simulink model "01_ee_a"  (R2023a)
settings: Solver=VariableStepDiscrete  StartTime=0.0  StopTime=6  RelTol=1e-3  EnableMultiTasking=on
PreLoadFcn:
  | %DFIG Data
  | clear;
  | NumberOfDFIG=100;
  | PnomDFIG=2e6*NumberOfDFIG; % Nominal power of DFIG(VA)
  | VnomDFIG=690;       % Line-Line voltage (Vrms)
  | fnom=50;
  | Rs=0.0108;     %pu
  | Lls=0.102;      %pu
  | Rr=0.01021;       %pu
  | Llr=0.11;      %pu
  | Lm=3.362;         %pu
  | Hg=2;         %Inertia constant (s)
  | F=0.01;         %Friction factor (pu)
  | p=2;            %Number of pairs of poles
  | kt=3;     %Rotor/Stator turns rotio
  | slip=-0.1;
  | 
  | %DC link
  | Vdc_nom=1200;       %Volts
  | C_DClink=15000e-6*NumberOfDFIG; %Farads
  | 
  | %Choke data
  | R_RL=0.15/100;  %pu
  | L_RL=0.15;      %pu
InitFcn:
  | Ts_Power = 10e-6;
  | Ts_Control = 100e-6;
  | PWM_freq=50*40;
undefined symbols (not defined in the file): D1, Delta, DiscIntNeverNeededParam
libraries: powerlib_extras x23, spsThreePhaseVIMeasurementLib x4, simulink_extras x4, spsThreePhaseTransformerTwoWindingsLib x2, spsUniversalBridgeLib x2, spsThreePhaseSeriesRLCBranchLib x2, spsParallelRLCBranchLib x1, spsThreePhaseProgrammableVoltageSourceLib x1, spsAsynchronousMachinepuUnitsLib x1, spsThreePhaseSeriesRLCLoadLib x1, spsGroundLib x1, spsMultimeterLib x1
(part 1 of 2)
settings Model: SimulationMode=accelerator  Creator=eagleyi  LastModifiedBy=eagle
settings SolverCC: AlgebraicLoopSolver=TrustRegion
settings DataIOCC: LimitDataPoints=on  SaveFormat=StructureWithTime  SignalLoggingSaveFormat=ModelDataLogs  ReturnWorkspaceOutputs=off
settings OptimizationCC: ExpressionDepthLimit=2147483647  InitFltsAndDblsToZero=on  LifeSpan=inf
settings DebuggingCC: UnderspecifiedInitializationDetection=Classic  MergeDetectMultiDrivingBlocksExec=none  SolverPrmCheckMsg=warning  FcnCallInpInsideContextMsg=warning  UnconnectedInputMsg=warning  UnconnectedOutputMsg=warning  UnconnectedLineMsg=warning  StateNameClashWarn=warning  SFUnexpectedBacktrackingDiag=warning  SFNoUnconditionalDefaultTransitionDiag=warning  SFExecutionAtInitializationDiag=none  ArithmeticOperatorsInVariantConditions=warning
settings HardwareCC: ProdBitPerPointer=32  ProdBitPerSizeT=32  ProdBitPerPtrDiffT=32  ProdLargestAtomicFloat=None  ProdIntDivRoundTo=Undefined  ProdEndianess=Unspecified  ProdWordSize=32  ProdHWDeviceType=32-bit Generic
settings ModelReferenceCC: PropagateSignalLabelsOutOfModel=off
settings SFSimCC: SimUseLocalCustomCode=off  CustomCodeUndefinedFunction=UseInterfaceOnly
settings RTWCC: RTWUseLocalCustomCode=off
settings CodeAppCC: StateflowObjectComments=on
settings GRTTargetCC: TargetLangStandard=C89/C90 (ANSI)  CombineOutputUpdateFcns=off  GRTInterface=on
settings ConfigComp: CovMetricSettings=dw  CovSaveCumulativeToWorkspaceVar=on  CovSaveSingleToWorkspaceVar=on  CovExternalEMLEnable=off  CovSFcnEnable=off
settings SimscapeCC: SimscapeNormalizeSystem=off

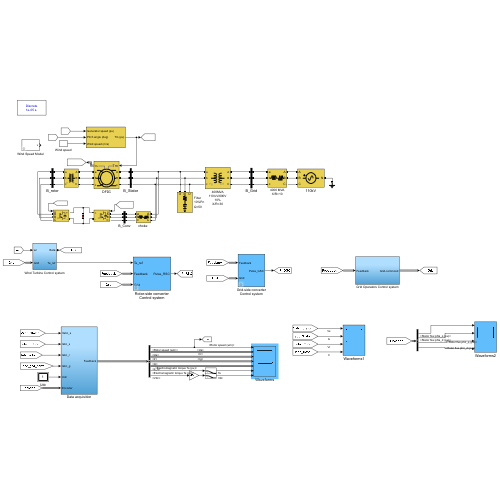
[thumbnail: Simulink's stored preview of the top-level diagram]
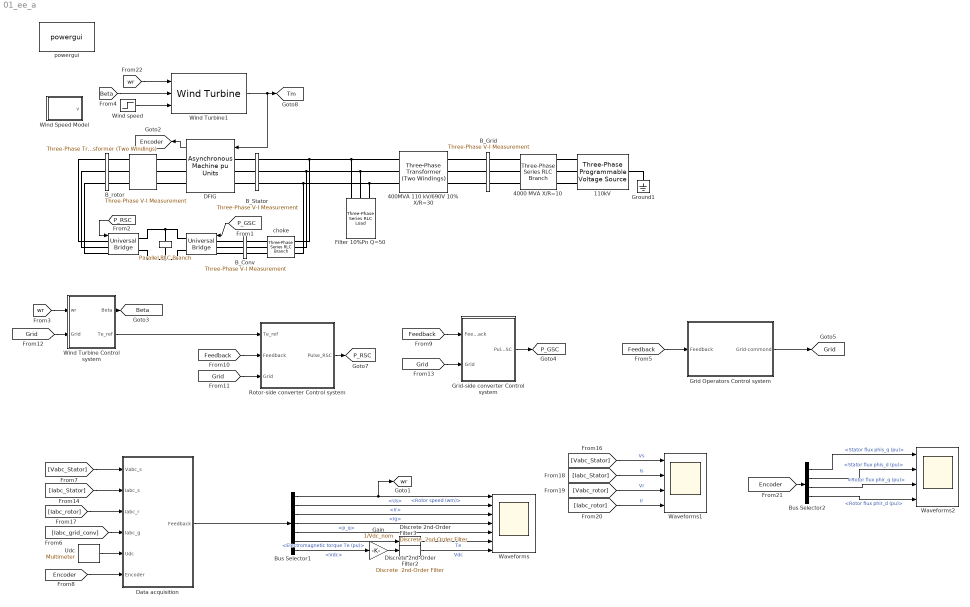
== system 01_ee_a ==
  " " : spsParallelRLCBranchLib/Parallel RLC Branch  LConnTagsString=a  RConnTagsString=__new0  BranchType=C  Resistance=1000  Inductance=1e-3  SetiL0=off  InitialCurrent=0  Capacitance=C_DClink  Setx0=on  InitialVoltage=Vdc_nom  Measurements=Branch voltage
  "  " : spsThreePhaseTransformerTwoWindingsLib/Three-Phase Transformer (Two Windings)  Winding1Connection=Y  Winding2Connection=Y  CoreType=Three single-phase transformers  SetSaturation=off  Hysteresis=off  DataFile='basic_model'  SetInitialFlux=off  Measurements=None  UNITS=pu  NominalPower=[PnomDFIG*0.3 5 ]  Winding1="[ VnomDFIG*0.25  0   0]"  Winding2="[VnomDFIG*0.25*kt  0  0.0001]"  Rm=500  Lm=500  L0=0.5  Saturation="[ 0,0  ;  0.005,1.2  ;  1.0,1.4 ]"  InitialFluxes=[ 0.8 , -0.8 , 0.7 ]  BreakLoop=off  DiscreteSolver=Trapezoidal iterative  DataType=off  TransfoNumber=0
  "   " : spsUniversalBridgeLib/Universal Bridge  Arms=3  SnubberResistance=1e5  SnubberCapacitance=inf  Device=IGBT / Diodes  Ron=1e-5  Lon=0  ForwardVoltages="[  0  0  ]"  ForwardVoltage=0  GTOparameters=[ 10e-6 , 20e-6 ]  IGBTparameters=[ 0 , 0 ]  Measurements=None  Measurements_2=None  converterType=Rectifier
  "          " : spsUniversalBridgeLib/Universal Bridge  Arms=3  SnubberResistance=1e5  SnubberCapacitance=inf  Device=IGBT / Diodes  Ron=1e-5  Lon=0  ForwardVoltages="[  0  0  ]"  ForwardVoltage=0  GTOparameters=[ 10e-6 , 20e-6 ]  IGBTparameters=[ 0 , 0 ]  Measurements=None  Measurements_2=None  converterType=Rectifier
  110kV : spsThreePhaseProgrammableVoltageSourceLib/Three-Phase Programmable Voltage Source  PositiveSequence=[110e3 0 fnom]  VariationEntity=Amplitude  VariationType=Table of time-amplitude pairs  VariationTypeAlt=Step  VariationStep=-0.2  VariationRate=10  VariationMagnitude=0.3  VariationFrequency=2  VariationTiming=[0.05 0.05+5/60]  VariationPhaseA=off  Amplitudes=[1 0.4 1.0]  TimeValues=[0 5 5.625]  HarmonicGeneration=off  HarmonicA=[1 0 0 2]  HarmonicB=[0 0 0 0]  Timing="[1  20]"  BusType=swing  Pref=0  Qref=0  Qmin=-inf  Qmax=inf
  4000 MVA X/R=10 : spsThreePhaseSeriesRLCBranchLib/Three-Phase Series RLC Branch  LConnTagsString=A|B|C  RConnTagsString=A|B|C  BranchType=RL  Resistance=0.1*110^2/4000  Inductance=1/(2*pi*50)*110^2/4000  Capacitance=1.0  Measurements=None
  400MVA 110 kV/690V 10% X/R=30 : spsThreePhaseTransformerTwoWindingsLib/Three-Phase Transformer (Two Windings)  Winding1Connection=Delta (D1)  Winding2Connection=Yg  CoreType=Three single-phase transformers  SetSaturation=off  Hysteresis=off  DataFile='basic_model'  SetInitialFlux=off  Measurements=None  UNITS=pu  NominalPower=[400e6 fnom ]  Winding1="[ 110e3  0.05/30   0.05]"  Winding2="[ 690 0.05/30  0.05]"  Rm=500  Lm=500  L0=0.5  Saturation="[ 0,0  ;  0.005,1.2  ;  1.0,1.4 ]"  InitialFluxes=[ 0.8 , -0.8 , 0.7 ]  BreakLoop=off  DiscreteSolver=Trapezoidal iterative  DataType=off  TransfoNumber=0
  B_Conv : spsThreePhaseVIMeasurementLib/Three-Phase V-I Measurement  VoltageMeasurement=no  SetLabelV=on  LabelV=Vabc_grid_conv  Vpu=off  VpuLL=off  CurrentMeasurement=yes  SetLabelI=on  LabelI=Iabc_grid_conv  Ipu=on  Pbase=PnomDFIG  Vbase=VnomDFIG  OutputType=Complex  PhasorSimulation=off  PSBequivalent=0
  B_Grid : spsThreePhaseVIMeasurementLib/Three-Phase V-I Measurement  VoltageMeasurement=no  SetLabelV=on  LabelV=Vabc_B6  Vpu=on  VpuLL=off  CurrentMeasurement=no  SetLabelI=on  LabelI=Iabc_B4  Ipu=on  Pbase=Pnom  Vbase=115e3  OutputType=Complex  PhasorSimulation=off  PSBequivalent=0
  B_Stator : spsThreePhaseVIMeasurementLib/Three-Phase V-I Measurement  VoltageMeasurement=phase-to-ground  SetLabelV=on  LabelV=Vabc_Stator  Vpu=on  VpuLL=off  CurrentMeasurement=yes  SetLabelI=on  LabelI=Iabc_Stator  Ipu=on  Pbase=PnomDFIG  Vbase=VnomDFIG  OutputType=Complex  PhasorSimulation=off  PSBequivalent=0
  B_rotor : spsThreePhaseVIMeasurementLib/Three-Phase V-I Measurement  VoltageMeasurement=phase-to-phase  SetLabelV=on  LabelV=Vabc_rotor  Vpu=on  VpuLL=off  CurrentMeasurement=yes  SetLabelI=on  LabelI=Iabc_rotor  Ipu=on  Pbase=PnomDFIG  Vbase=VnomDFIG*3  OutputType=Complex  PhasorSimulation=off  PSBequivalent=0
  Bus Selector1 : BusSelector  OutputSignals=Power&Torque&Speed.Rotor speed (wm),Synchronous Frame.Us,Synchronous Frame.Ir,Synchronous Frame.Ig,Power&Torque&Speed.p&q_stator.p_q,Power&Torque&Speed.Electromagnetic torque Te (pu),Stationary Frame.Vdc
  Bus Selector2 : BusSelector  OutputSignals=Stator measurements.Stator flux phis_q (pu),Stator measurements.Stator flux phis_d (pu),Rotor measurements.Rotor flux phir_q (pu),Rotor measurements.Rotor flux phir_d (pu)
  DFIG : spsAsynchronousMachinepuUnitsLib/Asynchronous Machine pu Units  RotorType=Wound  PresetModel=No  MechanicalLoad=Torque Tm  ShowDetailedParameters=on  ReferenceFrame=Synchronous  Units=pu  MeasurementBus=off  NominalParameters=[PnomDFIG VnomDFIG fnom]  VoltageRatio=1  Stator=[Rs Lls]  Rotor=[Rr Llr]  Cage1=[0.01909 0.0397]  Cage2=[0.01909 0.0397]  Lm=Lm  Mechanical=[Hg F p]  PolePairs=2  InitialConditions="[ slip, 0   0,0,0   0,0,0 ]"  SimulateSaturation=off  Saturation="[0.212,0.4201,0.8125,1.0979,1.4799,2.2457,3.2586,4.5763,6.4763 ;   0.5,0.7,0.9,1,1.1,1.2 ,1.3,1.4,1.5]"  LoadFlowParameters=0  TsPowergui=0  TsBlock=-1  IterativeModel=Forward Euler  IterativeDiscreteModel=Trapezoidal non iterative  Pmec=0
      settings: LibrarySourceBlock=|
      | sps_lib/Electrical Machines/Asynchronous Machine
      | pu Units
  Data acquisition : Subsystem
  Discrete 2nd-Order Filter2 : powerlib_extras/Discrete  Control Blocks/Discrete  2nd-Order Filter  FilterType=Lowpass  Fo=1000  Zeta=0.707  Ts=Ts_Power  Initialize=off  Vac_Init=[0.8 -25 60]  Vdc_Init=-0.4  PlotResponse=off  param1=[1 5000 10]
  Discrete 2nd-Order Filter3 : powerlib_extras/Discrete  Control Blocks/Discrete  2nd-Order Filter  FilterType=Lowpass  Fo=1000  Zeta=0.707  Ts=Ts_Power  Initialize=off  Vac_Init=[0.8 -25 60]  Vdc_Init=-0.4  PlotResponse=off  param1=[1 5000 10]
  Filter 10%Pn Q=50 : spsThreePhaseSeriesRLCLoadLib/Three-Phase Series RLC Load  LConnTagsString=A|B|C  Configuration=Y (grounded)  NominalVoltage=VnomDFIG  Vabc=[1e3 1e3 1e3]  Vabcp=[1e3 1e3 1e3]  NominalFrequency=fnom  UnbalancedPower=off  ActivePower=PnomDFIG*0.1/50  InductivePower=0  CapacitivePower=PnomDFIG*0.1  Pabc=[10e3 9e3 11e3]  QLabc=[100 90 110]  QCabc=[100 90 110]  Pabcp=[10e3 9e3 11e3]  QLabcp=[100 90 110]  QCabcp=[100 90 110]  Measurements=None  LoadType=constant Z
  Gain : Gain  Gain=1/Vdc_nom
  Grid Operators Control system : Subsystem
  Grid-side converter Control system : Subsystem  mask{Kpi_grid_side=[0.5 100 1], Kpi_DC_voltage=[2 20 0.5]}
      mask prompts: Kpi_grid_side "PI controller of Grid-side Current"; Kpi_DC_voltage "PI controller of DC Voltage"
      mask init:
      | Kp_grid_side_cur_reg=Kpi_grid_side(1);
      | Ki_grid_side_cur_reg=Kpi_grid_side(2);
      | Limit_U_grid_side=Kpi_grid_side(3);
      | Kp_dc_reg=Kpi_DC_voltage(1);
      | Ki_dc_reg=Kpi_DC_voltage(2);
      | Imax_grid_conv=Kpi_DC_voltage(3);
  Ground1 : spsGroundLib/Ground  LConnTagsString=a
  Rotor-side converter Control system : Subsystem  mask{KQ=[0.5 100 1], K_Irp=[0.5 100 1]}
      mask prompts: KQ "Reactive Power Controller [Kp Ki Limit]"; K_Irp "Rotor Curretnt Controller [Kp Ki Limit]"
      mask init:
      | Kp_Q=KQ(1);
      | Ki_Q=KQ(2);
      | Limit_Q=KQ(3);
      | Kp_rotor_side_cur_reg_P=K_Irp(1);
      | Ki_rotor_side_cur_reg_P=K_Irp(2);
      | Limit_U=K_Irp(3);
  Udc : spsMultimeterLib/Multimeter  L=1  sel=1  yselected={}  Gain=1  OutputType=Complex  PlotAtSimulationStop=off  PhasorSimulation=off
  Waveforms : Scope  NumInputPorts=7
  Waveforms1 : Scope  NumInputPorts=4
  Waveforms2 : Scope  NumInputPorts=4
  Wind Speed Model : Subsystem  mask{Vav=8, Vte=[5 10 3], Vgr=[5 35 2], Vnmax=1}
      mask prompts: Vav "Average wind speed"; Vte "Terbulent wind [tg1  Tg  Vgmax]"; Vgr "Gradual wind [tr1 tr2 Vrmax]"; Vnmax "Random wind Vrmax"
      mask init:
      | tg1=Vte(1);
      | Tg=Vte(2);
      | Vgmax=Vte(3);
      | tr1=Vgr(1);
      | tr2=Vgr(2);
      | Vrmax=Vgr(3);
  Wind Turbine Control system : Subsystem
  Wind Turbine1 : spsWindTurbineLib/Wind Turbine  Pnom=PnomDFIG  Pelec_base=PnomDFIG  wind_base=12  P_wind_base=1  speed_nom=1.1  pitch_angle=0  c1_c6="[0.51763          116          0.4            5           21     0.006795]"  cp_nom=0.48  lambda_nom=8.1
  Wind speed : Step  Time=4  Before=12  After=12  SampleTime=0
  "choke " : spsThreePhaseSeriesRLCBranchLib/Three-Phase Series RLC Branch  LConnTagsString=A|B|C  RConnTagsString=A|B|C  BranchType=RL  Resistance=R_RL*VnomDFIG^2/(0.1*PnomDFIG)  Inductance=L_RL*VnomDFIG^2/(0.1*PnomDFIG)/(2*pi*fnom)  Capacitance=[]  Measurements=None
  powergui : sps_lib/powergui  Priority=2  SimulationMode=Discrete  SampleTime=Ts_Power  frequency=60  Iterations=50  frequencyindice=0  Pbase=100e6  ErrMax=1e-4  UnitsV=kV  UnitsW=MW  buscounter=0  FunctionMessages=off  echomessages=on  EnableUseOfTLC=off  CurrentSourceSwitches=off  DisableSnubberDevices=off  DisableRonSwitches=off  DisableVfSwitches=off  DisplayEquations=off  AutomaticDiscreteSolvers=off  SolverType=Tustin  Interpol=off  ExternalGateDelay=off  methode=off  Ts=0  x0status=blocks  SPID=off  SwTol=0  HookPort=off  NonlinearTolerance=1e-4  nMaxIteration=100  ContinueOnMaxIteration=off  RestoreLinks=warning  ResistiveCurrentMeasurement=off  Frange=[0:2:500]  Ylog=off  Xlog=on  ShowGrid=off  save=off  variable=ZData  structure=ScopeData1  ZoomFFT=off  StartTime=1.4  cycles=1  DisplayStyle=1  fundamental=50  FreqAxis=off  MaxFrequency=500  frequencyindicesteady=1  RmsSteady=1  display=off
  tag scope: Beta=global, Encoder=global, Grid=global, P_GSC=global, P_RSC=global, Tm=global, wr=global
  wires:
  DFIG/1 -> [Encoder]
  [P_GSC] -> "          "/1
  [P_RSC] -> "   "/1
  Bus Selector1/4 -> Waveforms/4  "<Ig>"
  Bus Selector1/1 -> [wr], Waveforms/1  "<Rotor speed (wm)>"
  Bus Selector1/2 -> Waveforms/2  "<Us>"
  Bus Selector1/3 -> Waveforms/3  "<Ir>"
  Bus Selector1/5 -> Waveforms/5  "<p_q>"
  Bus Selector1/6 -> Discrete 2nd-Order Filter2/1  "<Electromagnetic torque Te (pu)>"
  Bus Selector1/7 -> Gain/1  "<Vdc>"
  Gain/1 -> Discrete 2nd-Order Filter3/1
  Discrete 2nd-Order Filter2/1 -> Waveforms/6  "Te"
  Discrete 2nd-Order Filter3/1 -> Waveforms/7  "Vdc"
  Wind Turbine Control system/1(Beta) -> [Beta]
  Grid-side converter Control system/1(Pulse_GSC) -> [P_GSC]
  [Vabc_Stator] -> Data acquisition/1(Vabc_s)
  [Iabc_Stator] -> Data acquisition/2(Iabc_s)
  [Iabc_rotor] -> Data acquisition/3(Iabc_r)
  Udc/1 -> Data acquisition/5(Udc)
  [Iabc_grid_conv] -> Data acquisition/4(Iabc_g)
  [Encoder] -> Data acquisition/6(Encoder)
  Data acquisition/1(Feedback) -> Bus Selector1/1
  Rotor-side converter Control system/1(Pulse_RSC) -> [P_RSC]
  Wind Turbine Control system/2(Te_ref) -> Rotor-side converter Control system/1(Te_ref)
  [Feedback] -> Grid-side converter Control system/1(Feedback)
  [Feedback] -> Rotor-side converter Control system/2(Feedback)
  [wr] -> Wind Turbine Control system/1(wr)
  [Grid] -> Rotor-side converter Control system/3(Grid)
  Grid Operators Control system/1(Grid-commond) -> [Grid]
  [Grid] -> Wind Turbine Control system/2(Grid)
  [Grid] -> Grid-side converter Control system/2(Grid)
  Wind Turbine1/1 -> DFIG/1, [Tm]
  [Feedback] -> Grid Operators Control system/1(Feedback)
  Wind speed/1 -> Wind Turbine1/3
  [Vabc_Stator] -> Waveforms1/1  "Vs"
  [Iabc_Stator] -> Waveforms1/2  "Is"
  [Vabc_rotor] -> Waveforms1/3  "Vr"
  [Iabc_rotor] -> Waveforms1/4  "Ir"
  [Encoder] -> Bus Selector2/1
  Bus Selector2/4 -> Waveforms2/4  "<Rotor flux phir_d (pu)>"
  Bus Selector2/1 -> Waveforms2/1  "<Stator flux phis_q (pu)>"
  Bus Selector2/2 -> Waveforms2/2  "<Stator flux phis_d (pu)>"
  Bus Selector2/3 -> Waveforms2/3  "<Rotor flux phir_q (pu)>"
  [wr] -> Wind Turbine1/1
  [Beta] -> Wind Turbine1/2
  connections:
  "   "/RConn1 -- " "/LConn1 -- "          "/RConn1
  "          "/RConn2 -- " "/RConn1 -- "   "/RConn2
  B_Stator/LConn1 -- Filter 10%Pn Q=50/LConn1 -- 400MVA 110 kV/690V 10% X/R=30/RConn1 -- "choke "/LConn1
  B_Stator/LConn2 -- Filter 10%Pn Q=50/LConn2 -- 400MVA 110 kV/690V 10% X/R=30/RConn2 -- "choke "/LConn2
  B_Stator/LConn3 -- Filter 10%Pn Q=50/LConn3 -- 400MVA 110 kV/690V 10% X/R=30/RConn3 -- "choke "/LConn3
  DFIG/LConn2 -- B_Stator/RConn2
  B_Conv/LConn2 -- "choke "/RConn2
  DFIG/LConn3 -- B_Stator/RConn3
  DFIG/LConn1 -- B_Stator/RConn1
  "          "/LConn3 -- B_Conv/RConn3
  B_Conv/LConn3 -- "choke "/RConn3
  "          "/LConn2 -- B_Conv/RConn2
  B_rotor/LConn2 -- "   "/LConn2
  B_rotor/LConn3 -- "   "/LConn3
  B_rotor/LConn1 -- "   "/LConn1
  "          "/LConn1 -- B_Conv/RConn1
  B_Conv/LConn1 -- "choke "/RConn1
  4000 MVA X/R=10/LConn1 -- 110kV/RConn1
  4000 MVA X/R=10/LConn2 -- 110kV/RConn2
  4000 MVA X/R=10/LConn3 -- 110kV/RConn3
  Ground1/LConn1 -- 110kV/LConn1
  B_Grid/LConn1 -- 4000 MVA X/R=10/RConn1
  B_Grid/LConn2 -- 4000 MVA X/R=10/RConn2
  B_Grid/LConn3 -- 4000 MVA X/R=10/RConn3
  400MVA 110 kV/690V 10% X/R=30/LConn1 -- B_Grid/RConn1
  400MVA 110 kV/690V 10% X/R=30/LConn2 -- B_Grid/RConn2
  400MVA 110 kV/690V 10% X/R=30/LConn3 -- B_Grid/RConn3
  "  "/LConn1 -- DFIG/RConn1
  "  "/LConn2 -- DFIG/RConn2
  "  "/LConn3 -- DFIG/RConn3
  B_rotor/RConn1 -- "  "/RConn1
  B_rotor/RConn2 -- "  "/RConn2
  B_rotor/RConn3 -- "  "/RConn3

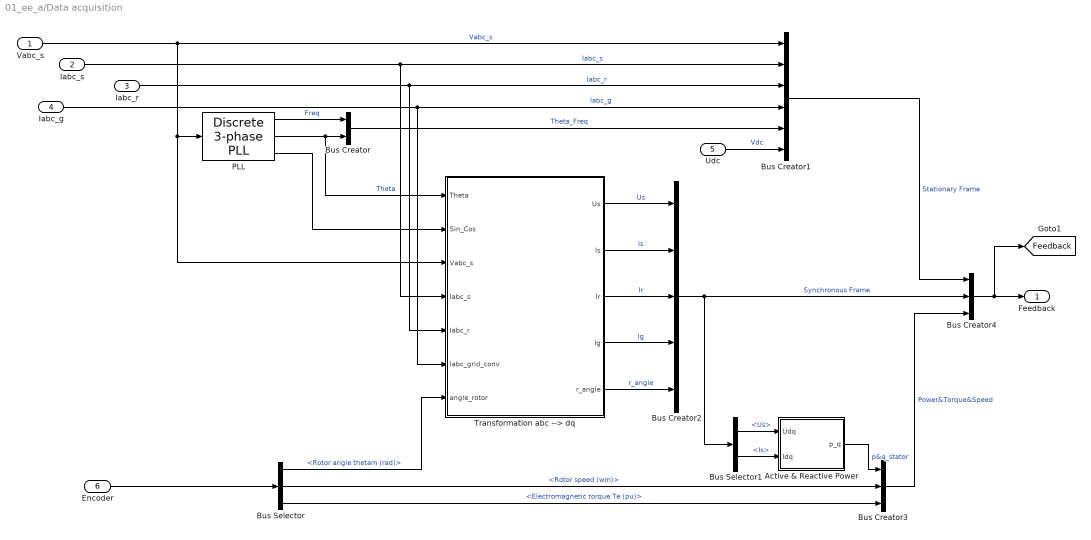
== system 01_ee_a/Data acquisition ==
  Vabc_s : Inport
  Iabc_s : Inport  Port=2
  Iabc_r : Inport  Port=3
  Iabc_g : Inport  Port=4
  Udc : Inport  Port=5
  Encoder : Inport  Port=6
  Active & Reactive Power : Subsystem
  Bus Creator : BusCreator  Inputs=2
  Bus Creator1 : BusCreator  Inputs=6
  Bus Creator2 : BusCreator  Inputs=5
  Bus Creator3 : BusCreator  Inputs=3
  Bus Creator4 : BusCreator  Inputs=3
  Bus Selector : BusSelector  OutputSignals=Mechanical.Rotor angle thetam (rad),Mechanical.Rotor speed (wm),Mechanical.Electromagnetic torque Te (pu)
  Bus Selector1 : BusSelector  OutputSignals=Us,Is
  PLL : powerlib_extras/Discrete  Control Blocks/Discrete 3-phase PLL  Fmin=45  Par_Init=[0 fnom]  ParK=[60 1400]  Ts=Ts_Power  AGC=off
  "Transformation abc --> dq " : Subsystem
  Feedback : Outport
  tag scope: Feedback=global
  wires:
  Encoder/1 -> Bus Selector/1
  Bus Selector/1 -> "Transformation abc --> dq "/7(angle_rotor)  "<Rotor angle thetam (rad)>"
  Vabc_s/1 -> Bus Creator1/1, "Transformation abc --> dq "/3(Vabc_s), PLL/1  "Vabc_s"
  Iabc_s/1 -> "Transformation abc --> dq "/4(Iabc_s), Bus Creator1/2  "Iabc_s"
  Iabc_r/1 -> "Transformation abc --> dq "/5(Iabc_r), Bus Creator1/3  "Iabc_r"
  Bus Creator/1 -> Bus Creator1/5  "Theta_Freq"
  Iabc_g/1 -> "Transformation abc --> dq "/6(Iabc_grid_conv), Bus Creator1/4  "Iabc_g"
  PLL/1 -> Bus Creator/1  "Freq"
  PLL/2 -> "Transformation abc --> dq "/1(Theta), Bus Creator/2  "Theta"
  PLL/3 -> "Transformation abc --> dq "/2(Sin_Cos)
  "Transformation abc --> dq "/1(Us) -> Bus Creator2/1  "Us"
  "Transformation abc --> dq "/5(r_angle) -> Bus Creator2/5  "r_angle"
  Udc/1 -> Bus Creator1/6  "Vdc"
  Bus Creator1/1 -> Bus Creator4/1  "Stationary Frame"
  Bus Creator2/1 -> Bus Selector1/1, Bus Creator4/2  "Synchronous Frame"
  Bus Creator3/1 -> Bus Creator4/3  "Power&Torque&Speed"
  Bus Creator4/1 -> Feedback/1, [Feedback]
  Active & Reactive Power/1(p_q) -> Bus Creator3/1  "p&q_stator"
  Bus Selector/2 -> Bus Creator3/2  "<Rotor speed (wm)>"
  Bus Selector/3 -> Bus Creator3/3  "<Electromagnetic torque Te (pu)>"
  Bus Selector1/1 -> Active & Reactive Power/1(Udq)  "<Us>"
  Bus Selector1/2 -> Active & Reactive Power/2(Idq)  "<Is>"
  "Transformation abc --> dq "/2(Is) -> Bus Creator2/2  "Is"
  "Transformation abc --> dq "/3(Ir) -> Bus Creator2/3  "Ir"
  "Transformation abc --> dq "/4(Ig) -> Bus Creator2/4  "Ig"

== system 01_ee_a/Grid Operators Control system ==
  Feedback : Inport
  Bus Creator1 : BusCreator  Inputs=4
  Bus Selector1 : BusSelector  OutputSignals=Synchronous Frame.Us.d
  Iq-ref : Step  Time=3  After=0.1  SampleTime=0
  Max Power : Constant
  Vdc_ref1 : Constant  Value=Vdc_nom
  Vs_ref : Constant
  voltage control : Subsystem
  Grid-commond : Outport
  wires:
  Vdc_ref1/1 -> Bus Creator1/1  "Vdc_nom"
  Iq-ref/1 -> Bus Creator1/2  "Qg_ref"
  Max Power/1 -> Bus Creator1/4  "Max Power"
  Bus Creator1/1 -> Grid-commond/1
  voltage control/1(Q_ref) -> Bus Creator1/3  "Qs_ref"
  Vs_ref/1 -> voltage control/1(Vs_ref)  "Vs_ref"
  Feedback/1 -> Bus Selector1/1
  Bus Selector1/1 -> voltage control/2(Us)  "<d>"

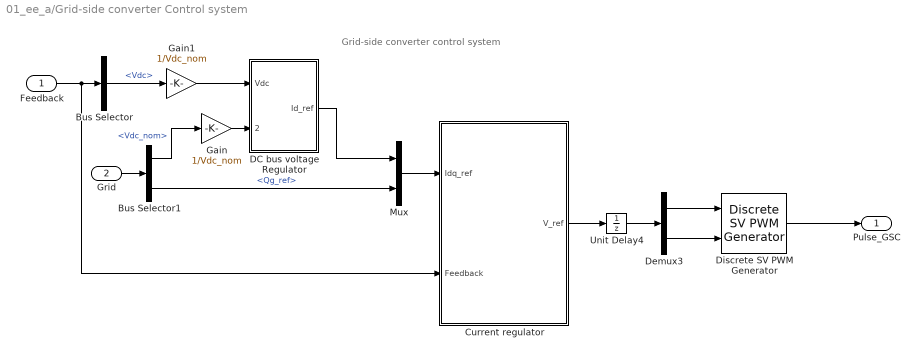
== system 01_ee_a/Grid-side converter Control system ==
  note: Grid-side converter control system
  Feedback : Inport
  Grid : Inport  Port=2
  Bus Selector : BusSelector  OutputSignals=Stationary Frame.Vdc
  Bus Selector1 : BusSelector  OutputSignals=Vdc_nom,Qg_ref
  Current regulator : Subsystem
  DC bus voltage Regulator : Subsystem
  Demux3 : Demux  Outputs=2
  Discrete SV PWM Generator : powerlib_extras/Discrete  Control Blocks/Discrete SV PWM Generator  InputType=alpha-beta components  SwitchingPattern=Pattern #1  Fc=PWM_freq  ParUref=[0.8 -30 50]  Ts=Ts_Power
  Gain : Gain  Gain=1/Vdc_nom
  Gain1 : Gain  Gain=1/Vdc_nom
  Mux : Mux  Inputs=2
  Unit Delay4 : UnitDelay  SampleTime=Ts_Power  HasFrameUpgradeWarning=on
  Pulse_GSC : Outport
  wires:
  Bus Selector/1 -> Gain1/1  "<Vdc>"
  DC bus voltage Regulator/1(Id_ref) -> Mux/1
  Mux/1 -> Current regulator/1(Idq_ref)
  Discrete SV PWM Generator/1 -> Pulse_GSC/1
  Feedback/1 -> Bus Selector/1, Current regulator/2(Feedback)
  Unit Delay4/1 -> Demux3/1
  Current regulator/1(V_ref) -> Unit Delay4/1
  Demux3/1 -> Discrete SV PWM Generator/1
  Demux3/2 -> Discrete SV PWM Generator/2
  Gain1/1 -> DC bus voltage Regulator/1(Vdc)
  Grid/1 -> Bus Selector1/1
  Gain/1 -> DC bus voltage Regulator/2(Vdc_ref)
  Bus Selector1/1 -> Gain/1  "<Vdc_nom>"
  Bus Selector1/2 -> Mux/2  "<Qg_ref>"

== system 01_ee_a/Rotor-side converter Control system ==
  Te_ref : Inport
  Feedback : Inport  Port=2
  Grid : Inport  Port=3
  Demux3 : Demux  Outputs=2
  Discrete SV PWM Generator : powerlib_extras/Discrete  Control Blocks/Discrete SV PWM Generator  InputType=alpha-beta components  SwitchingPattern=Pattern #1  Fc=PWM_freq  ParUref=[0.8 -30 50]  Ts=Ts_Power
  Inner loop control : Subsystem
  Outer loop control : Subsystem
  Unit Delay1 : UnitDelay  SampleTime=Ts_Power  HasFrameUpgradeWarning=on
  Pulse_RSC : Outport
  wires:
  Feedback/1 -> Inner loop control/2(Feedback), Outer loop control/3(Feedback)
  Outer loop control/1(Idqr_ref) -> Inner loop control/1(Idqr_ref)
  Discrete SV PWM Generator/1 -> Pulse_RSC/1
  Unit Delay1/1 -> Demux3/1
  Demux3/1 -> Discrete SV PWM Generator/1
  Demux3/2 -> Discrete SV PWM Generator/2
  Inner loop control/1(Uabc_ref) -> Unit Delay1/1
  Te_ref/1 -> Outer loop control/1(Te_ref)
  Grid/1 -> Outer loop control/2(Grid)

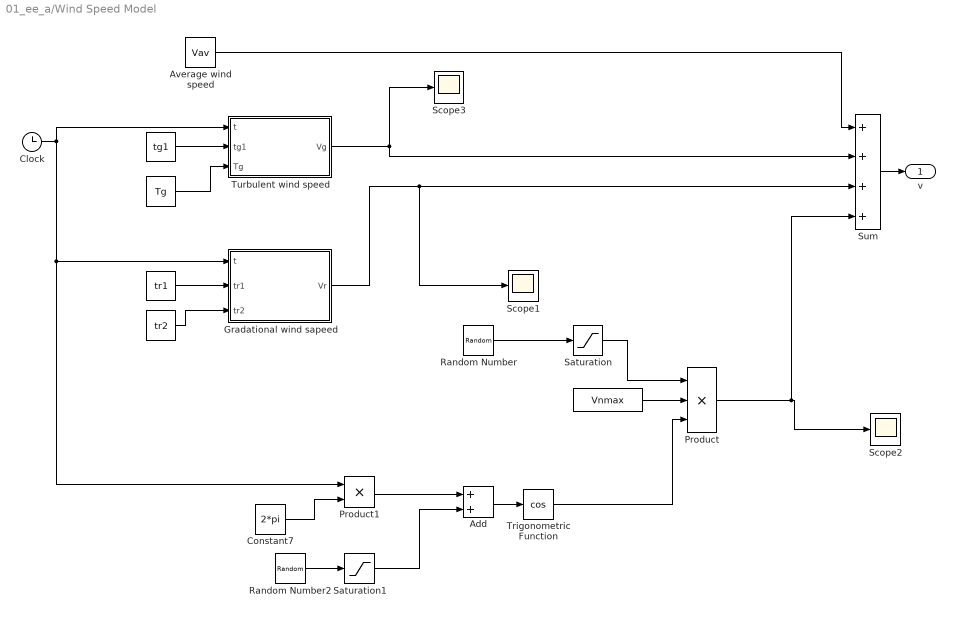
== system 01_ee_a/Wind Speed Model ==
  " " : Constant  Value=tg1
  "  " : Constant  Value=Tg
  "   " : Constant  Value=Vnmax
  "    " : Constant  Value=tr2
  "      " : Constant  Value=tr1
  Add : Sum
  Average wind speed : Constant  Value=Vav
  Clock : Clock
  Constant7 : Constant  Value=2*pi
  Gradational wind sapeed : Subsystem
  Product : Product  Inputs=3  RndMeth=Zero
  Product1 : Product  RndMeth=Zero
  Random Number : RandomNumber  Variance=0.1  SampleTime=1
  Random Number2 : RandomNumber  Mean=pi  Variance=0.1  SampleTime=1
  Saturation : Saturate  UpperLimit=1  LowerLimit=-1
  Saturation1 : Saturate  UpperLimit=2*pi  LowerLimit=0
  Scope1 : Scope
  Scope2 : Scope
  Scope3 : Scope
  Sum : Sum  Inputs=++++
  Trigonometric Function : Trigonometry  Operator=cos
  "Turbulent wind speed " : Subsystem
  v : Outport
  wires:
  Trigonometric Function/1 -> Product/3
  Add/1 -> Trigonometric Function/1
  Product1/1 -> Add/1
  Constant7/1 -> Product1/2
  "   "/1 -> Product/2
  "  "/1 -> "Turbulent wind speed "/3(Tg)
  "    "/1 -> Gradational wind sapeed/3(tr2)
  "      "/1 -> Gradational wind sapeed/2(tr1)
  Gradational wind sapeed/1(Vr) -> Sum/3, Scope1/1
  Clock/1 -> Product1/1, Gradational wind sapeed/1(t), "Turbulent wind speed "/1(t)
  "Turbulent wind speed "/1(Vg) -> Sum/2, Scope3/1
  Average wind speed/1 -> Sum/1
  " "/1 -> "Turbulent wind speed "/2(tg1)
  Sum/1 -> v/1
  Random Number/1 -> Saturation/1
  Random Number2/1 -> Saturation1/1
  Saturation/1 -> Product/1
  Saturation1/1 -> Add/2
  Product/1 -> Sum/4, Scope2/1

== system 01_ee_a/Wind Turbine Control system ==
  wr : Inport
  Grid : Inport  Port=2
  MPPT : Subsystem
  Pitch control : Subsystem
  Beta : Outport
  Te_ref : Outport  Port=2
  wires:
  wr/1 -> MPPT/1(wr), Pitch control/1(wr)
  Pitch control/1(Pitch angle) -> Beta/1
  MPPT/1(Te_ref) -> Te_ref/1
  Grid/1 -> MPPT/2(Grid)

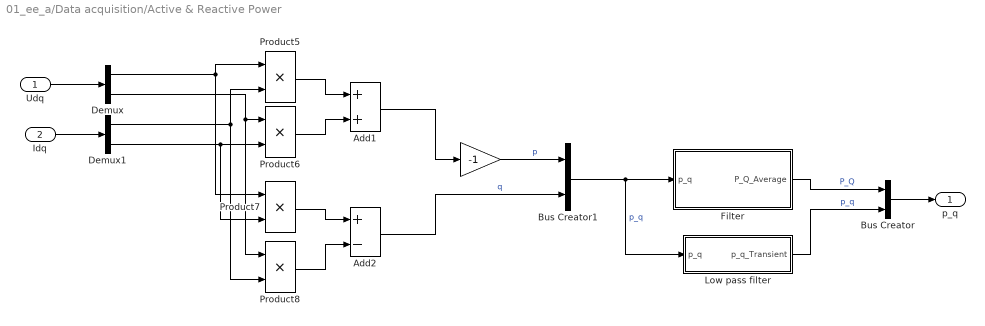
== system 01_ee_a/Data acquisition/Active & Reactive Power ==
  Udq : Inport
  Idq : Inport  Port=2
  "  " : Gain  Gain=-1  SaturateOnIntegerOverflow=on  OutDataTypeStr=Inherit: Same as input  ParamDataTypeStr=Inherit: Same as input
  Add1 : Sum
  Add2 : Sum  Inputs=+-
  Bus Creator : BusCreator  Inputs=2
  Bus Creator1 : BusCreator  Inputs=2
  Demux : Demux  Outputs=2
  Demux1 : Demux  Outputs=2
  Filter : Subsystem
  Low pass filter : Subsystem
  Product{5..8} (4 alike) : Product  InputSameDT=on  SaturateOnIntegerOverflow=on  OutDataTypeStr=Inherit: Same as first input
  p_q : Outport
  wires:
  Product5/1 -> Add1/1
  Product6/1 -> Add1/2
  Product7/1 -> Add2/1
  Product8/1 -> Add2/2
  Add2/1 -> Bus Creator1/2  "q"
  Add1/1 -> "  "/1
  Bus Creator1/1 -> Filter/1(p_q), Low pass filter/1(p_q)  "p_q"
  Udq/1 -> Demux/1
  Demux/1 -> Product5/1, Product7/1
  Idq/1 -> Demux1/1
  Demux1/1 -> Product5/2, Product8/2
  Demux/2 -> Product6/1, Product8/1
  Demux1/2 -> Product6/2, Product7/2
  "  "/1 -> Bus Creator1/1  "p"
  Bus Creator/1 -> p_q/1
  Filter/1(P_Q_Average) -> Bus Creator/1  "P_Q"
  Low pass filter/1("p_q_Transient ") -> Bus Creator/2  "p_q"

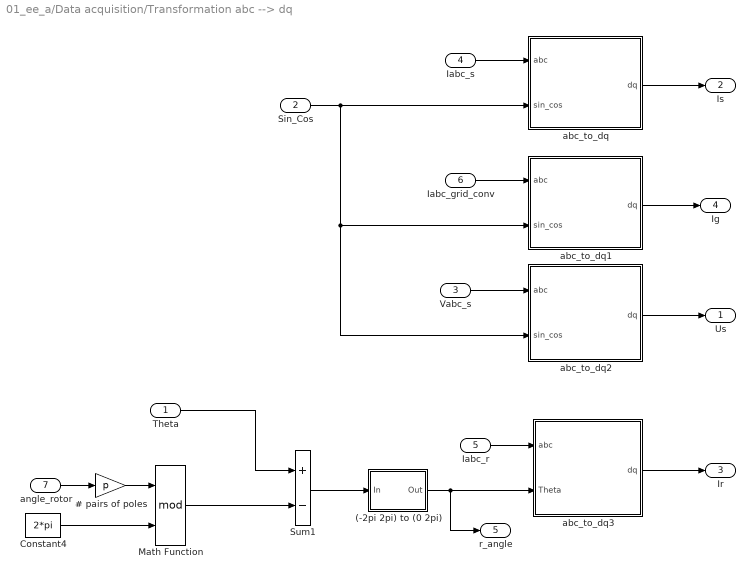
== system 01_ee_a/Data acquisition/Transformation abc --> dq  ==
  Theta : Inport
  Sin_Cos : Inport  Port=2
  Vabc_s : Inport  Port=3
  Iabc_s : Inport  Port=4
  Iabc_r : Inport  Port=5
  Iabc_grid_conv : Inport  Port=6
  angle_rotor : Inport  Port=7
  # pairs of poles : Gain  Gain=p  SaturateOnIntegerOverflow=on  OutDataTypeStr=Inherit: Same as input  ParamDataTypeStr=Inherit: Same as input
  (-2pi 2pi) to (0 2pi) : Subsystem
  Constant4 : Constant  Value=2*pi
  Math Function : Math  Operator=mod  SignedPower=on
  Sum1 : Sum  Inputs=+-  InputSameDT=on  SaturateOnIntegerOverflow=on  OutDataTypeStr=Inherit: Same as first input
  abc_to_dq : Subsystem
  abc_to_dq1 : Subsystem
  abc_to_dq2 : Subsystem
  abc_to_dq3 : Subsystem
  Us : Outport
  Is : Outport  Port=2
  Ir : Outport  Port=3
  Ig : Outport  Port=4
  r_angle : Outport  Port=5
  wires:
  angle_rotor/1 -> # pairs of poles/1
  Theta/1 -> Sum1/1
  Sum1/1 -> (-2pi 2pi) to (0 2pi)/1(In)
  Constant4/1 -> Math Function/2
  # pairs of poles/1 -> Math Function/1
  Math Function/1 -> Sum1/2
  Iabc_s/1 -> abc_to_dq/1(abc)
  Iabc_r/1 -> abc_to_dq3/1(abc)
  Vabc_s/1 -> abc_to_dq2/1(abc)
  Iabc_grid_conv/1 -> abc_to_dq1/1(abc)
  Sin_Cos/1 -> abc_to_dq/2(sin_cos), abc_to_dq1/2(sin_cos), abc_to_dq2/2(sin_cos)
  (-2pi 2pi) to (0 2pi)/1(Out) -> r_angle/1, abc_to_dq3/2(Theta)
  abc_to_dq2/1(dq) -> Us/1
  abc_to_dq/1(dq) -> Is/1
  abc_to_dq3/1(dq) -> Ir/1
  abc_to_dq1/1(dq) -> Ig/1

== system 01_ee_a/Grid Operators Control system/voltage control ==
  Vs_ref : Inport
  Us : Inport  Port=2
  Discrete PI Controller2 : Subsystem  AncestorBlock=|  DialogController=POWERSYS.PowerSysDialog  mask(Discrete PI Controller){Kp=1, Ki=5, Par_Limits=[1 -1]*0.5, Init=0, Ts=Ts_Control}
      | powerlib_extras/Discrete 
      | Control Blocks/Discrete
      | PI Controller
      mask prompts: Kp "Proportional gain (Kp):"; Ki "Integral gain (Ki):"; Par_Limits "Output limits: [ Upper   Lower ]"; Init "Output initial value:"; Ts "Sample time:"
      mask help: This block implements a discrete PI controller.
      mask init:
      | UpperLimit=Par_Limits(1);
      | LowerLimit=Par_Limits(2);
      | power_initmask();
      mask Help: This block is part of a subset of blocks in the Extras library that does not have documentation associated with it, other than the block mask description.
      mask Display: disp('PI');
  Discrete 2nd-Order Filter4 : powerlib_extras/Discrete  Control Blocks/Discrete  2nd-Order Filter  FilterType=Lowpass  Fo=50  Zeta=0.707  Ts=Ts_Power  Initialize=off  Vac_Init=[0.8 -25 60]  Vdc_Init=-0.4  PlotResponse=off  param1=[1 5000 10]
  Sum7 : Sum  Inputs=+-  InputSameDT=on  SaturateOnIntegerOverflow=on  OutDataTypeStr=Inherit: Same as first input
  Q_ref : Outport
  wires:
  Sum7/1 -> Discrete PI Controller2/1(Error)
  Discrete PI Controller2/1(Out) -> Q_ref/1
  Us/1 -> Discrete 2nd-Order Filter4/1
  Vs_ref/1 -> Sum7/1
  Discrete 2nd-Order Filter4/1 -> Sum7/2

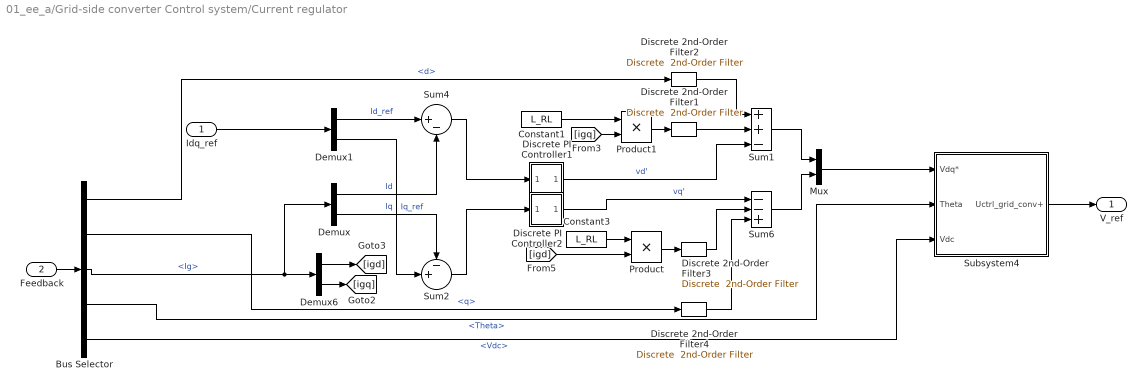
== system 01_ee_a/Grid-side converter Control system/Current regulator ==
  Idq_ref : Inport
  Feedback : Inport  Port=2
  Bus Selector : BusSelector  OutputSignals=Synchronous Frame.Us.d,Synchronous Frame.Us.q,Synchronous Frame.Ig,Stationary Frame.Theta_Freq.Theta,Stationary Frame.Vdc
  Constant1 : Constant  Value=L_RL
  Constant3 : Constant  Value=L_RL
  Demux : Demux  Outputs=2
      settings: DisplayOption=none
  Demux1 : Demux  Outputs=2
      settings: DisplayOption=none
  Demux6 : Demux  Outputs=2
      settings: DisplayOption=none
  Discrete PI Controller1 : Subsystem  AncestorBlock=|  DialogController=POWERSYS.PowerSysDialog  mask(Discrete PI Controller){Kp=Kp_grid_side_cur_reg, Ki=Ki_grid_side_cur_reg, Par_Limits=[1 -1]*Limit_U_grid_side, Init=0, Ts=Ts_Control}
      | powerlib_extras/Discrete 
      | Control Blocks/Discrete
      | PI Controller
      mask prompts: Kp "Proportional gain (Kp):"; Ki "Integral gain (Ki):"; Par_Limits "Output limits: [ Upper   Lower ]"; Init "Output initial value:"; Ts "Sample time:"
      mask help: This block implements a discrete PI controller.
      mask init:
      | UpperLimit=Par_Limits(1);
      | LowerLimit=Par_Limits(2);
      | power_initmask();
      mask Help: This block is part of a subset of blocks in the Extras library that does not have documentation associated with it, other than the block mask description.
      mask Display: disp('PI');
  Discrete PI Controller2 : Subsystem  AncestorBlock=|  DialogController=POWERSYS.PowerSysDialog  mask(Discrete PI Controller){Kp=Kp_grid_side_cur_reg*3, Ki=Ki_grid_side_cur_reg, Par_Limits=[1 -1]*Limit_U_grid_side, Init=0, Ts=Ts_Control}
      | powerlib_extras/Discrete 
      | Control Blocks/Discrete
      | PI Controller
      mask prompts: Kp "Proportional gain (Kp):"; Ki "Integral gain (Ki):"; Par_Limits "Output limits: [ Upper   Lower ]"; Init "Output initial value:"; Ts "Sample time:"
      mask help: This block implements a discrete PI controller.
      mask init:
      | UpperLimit=Par_Limits(1);
      | LowerLimit=Par_Limits(2);
      | power_initmask();
      mask Help: This block is part of a subset of blocks in the Extras library that does not have documentation associated with it, other than the block mask description.
      mask Display: disp('PI');
  Discrete 2nd-Order Filter{1..4} (4 alike) : powerlib_extras/Discrete  Control Blocks/Discrete  2nd-Order Filter  FilterType=Lowpass  Fo=50  Zeta=0.707  Ts=Ts_Power  Initialize=off  Vac_Init=[0.8 -25 60]  Vdc_Init=-0.4  PlotResponse=off  param1=[1 5000 10]
  Mux : Mux  Inputs=2
  Product : Product  RndMeth=Zero
  Product1 : Product  RndMeth=Zero
  Subsystem4 : Subsystem
  Sum1 : Sum  Inputs=++-  InputSameDT=on  SaturateOnIntegerOverflow=on  OutDataTypeStr=Inherit: Same as first input
  Sum2 : Sum  Inputs=-+|  InputSameDT=on  SaturateOnIntegerOverflow=on  OutDataTypeStr=Inherit: Same as first input
  Sum4 : Sum  Inputs=|+-  InputSameDT=on  SaturateOnIntegerOverflow=on  OutDataTypeStr=Inherit: Same as first input
  Sum6 : Sum  Inputs=--+  InputSameDT=on  SaturateOnIntegerOverflow=on  OutDataTypeStr=Inherit: Same as first input
  V_ref : Outport
  wires:
  Demux1/2 -> Sum2/2  "Iq_ref"
  Demux1/1 -> Sum4/1  "Id_ref"
  Demux/2 -> Sum2/1  "Iq"
  Demux/1 -> Sum4/2  "Id"
  Sum1/1 -> Mux/1
  Discrete PI Controller2/1(Out) -> Sum6/1  "vq'"
  Sum4/1 -> Discrete PI Controller1/1(Error)
  Sum2/1 -> Discrete PI Controller2/1(Error)
  Feedback/1 -> Bus Selector/1
  Bus Selector/4 -> Subsystem4/2(Theta)  "<Theta>"
  Sum6/1 -> Mux/2
  Discrete PI Controller1/1(Out) -> Sum1/3  "vd'"
  Mux/1 -> Subsystem4/1(Vdq*)
  Idq_ref/1 -> Demux1/1
  Constant1/1 -> Product1/1
  [igq] -> Product1/2
  Constant3/1 -> Product/1
  [igd] -> Product/2
  Product/1 -> Discrete 2nd-Order Filter3/1
  Bus Selector/5 -> Subsystem4/3(Vdc)  "<Vdc>"
  Product1/1 -> Discrete 2nd-Order Filter1/1
  Bus Selector/1 -> Discrete 2nd-Order Filter2/1  "<d>"
  Bus Selector/2 -> Discrete 2nd-Order Filter4/1  "<q>"
  Bus Selector/3 -> Demux6/1, Demux/1  "<Ig>"
  Demux6/1 -> [igd]
  Demux6/2 -> [igq]
  Subsystem4/1(Uctrl_grid_conv+) -> V_ref/1
  Discrete 2nd-Order Filter2/1 -> Sum1/1
  Discrete 2nd-Order Filter1/1 -> Sum1/2
  Discrete 2nd-Order Filter3/1 -> Sum6/2
  Discrete 2nd-Order Filter4/1 -> Sum6/3

== system 01_ee_a/Grid-side converter Control system/DC bus voltage Regulator ==
  Vdc : Inport
  Vdc_ref : Inport  Port=2
  Discrete PI Controller : Subsystem  AncestorBlock=|  DialogController=POWERSYS.PowerSysDialog  mask(Discrete PI Controller){Kp=Kp_dc_reg, Ki=Ki_dc_reg, Par_Limits=[1 -1]*Imax_grid_conv, Init=0, Ts=Ts_Control}
      | powerlib_extras/Discrete 
      | Control Blocks/Discrete
      | PI Controller
      mask prompts: Kp "Proportional gain (Kp):"; Ki "Integral gain (Ki):"; Par_Limits "Output limits: [ Upper   Lower ]"; Init "Output initial value:"; Ts "Sample time:"
      mask help: This block implements a discrete PI controller.
      mask init:
      | UpperLimit=Par_Limits(1);
      | LowerLimit=Par_Limits(2);
      | power_initmask();
      mask Help: This block is part of a subset of blocks in the Extras library that does not have documentation associated with it, other than the block mask description.
      mask Display: disp('PI');
  Sum7 : Sum  Inputs=|+-  InputSameDT=on  SaturateOnIntegerOverflow=on  OutDataTypeStr=Inherit: Same as first input
  Id_ref : Outport
  wires:
  Sum7/1 -> Discrete PI Controller/1(Error)
  Vdc_ref/1 -> Sum7/1
  Vdc/1 -> Sum7/2
  Discrete PI Controller/1(Out) -> Id_ref/1

== system 01_ee_a/Rotor-side converter Control system/Inner loop control ==
  Idqr_ref : Inport
  Feedback : Inport  Port=2
  Bus Selector1 : BusSelector  OutputSignals=Synchronous Frame.Is,Power&Torque&Speed.Rotor speed (wm),Stationary Frame.Theta_Freq.Freq,Synchronous Frame.Ir,Synchronous Frame.r_angle,Stationary Frame.Vdc
  Current Regulator : Subsystem
  Subsystem2 : Subsystem
  Uabc_ref : Outport
  wires:
  Bus Selector1/1 -> Current Regulator/2(Idq_s)  "<Is>"
  Bus Selector1/2 -> Current Regulator/3(wr)  "<Rotor speed (wm)>"
  Bus Selector1/3 -> Current Regulator/4(Freq)  "<Freq>"
  Idqr_ref/1 -> Current Regulator/1(Idqr+_ref)  "Idqr+_ref"
  Feedback/1 -> Bus Selector1/1
  Current Regulator/1(Vdq*) -> Subsystem2/1(Vdq*)  "Udq+_ref"
  Bus Selector1/5 -> Subsystem2/2(Theta)  "<r_angle>"
  Bus Selector1/6 -> Subsystem2/3(Vdc)  "<Vdc>"
  Bus Selector1/4 -> Current Regulator/5(Idq_r)  "<Ir>"
  Subsystem2/1(Uctrl_grid_conv1) -> Uabc_ref/1

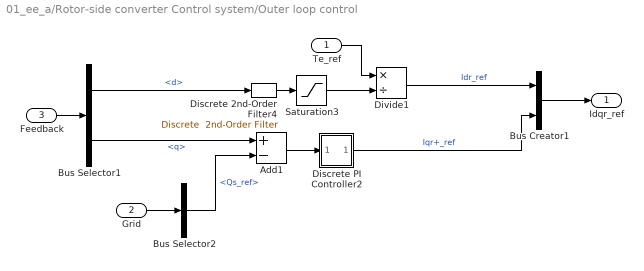
== system 01_ee_a/Rotor-side converter Control system/Outer loop control ==
  Te_ref : Inport
  Grid : Inport  Port=2
  Feedback : Inport  Port=3
  Add1 : Sum  Inputs=+-
  Bus Creator1 : BusCreator  Inputs=2
  Bus Selector1 : BusSelector  OutputSignals=Synchronous Frame.Us.d,Synchronous Frame.Is.q
  Bus Selector2 : BusSelector  OutputSignals=Qs_ref
  Discrete PI Controller2 : Subsystem  AncestorBlock=|  DialogController=POWERSYS.PowerSysDialog  mask(Discrete PI Controller){Kp=Kp_Q, Ki=Ki_Q, Par_Limits=[Limit_Q -Limit_Q ], Init=0, Ts=Ts_Control}
      | powerlib_extras/Discrete 
      | Control Blocks/Discrete
      | PI Controller
      mask prompts: Kp "Proportional gain (Kp):"; Ki "Integral gain (Ki):"; Par_Limits "Output limits: [ Upper   Lower ]"; Init "Output initial value:"; Ts "Sample time:"
      mask help: This block implements a discrete PI controller.
      mask init:
      | UpperLimit=Par_Limits(1);
      | LowerLimit=Par_Limits(2);
      | power_initmask();
      mask Help: This block is part of a subset of blocks in the Extras library that does not have documentation associated with it, other than the block mask description.
      mask Display: disp('PI');
  Discrete 2nd-Order Filter4 : powerlib_extras/Discrete  Control Blocks/Discrete  2nd-Order Filter  FilterType=Lowpass  Fo=50  Zeta=0.707  Ts=Ts_Power  Initialize=off  Vac_Init=[0.8 -25 60]  Vdc_Init=-0.4  PlotResponse=off  param1=[1 5000 10]
  Divide1 : Product  Inputs=*/
  Saturation3 : Saturate  UpperLimit=1.3  LowerLimit=0.7
  Idqr_ref : Outport
  wires:
  Add1/1 -> Discrete PI Controller2/1(Error)
  Feedback/1 -> Bus Selector1/1
  Bus Creator1/1 -> Idqr_ref/1
  Discrete PI Controller2/1(Out) -> Bus Creator1/2  "Iqr+_ref"
  Divide1/1 -> Bus Creator1/1  "Idr_ref"
  Bus Selector1/1 -> Discrete 2nd-Order Filter4/1  "<d>"
  Discrete 2nd-Order Filter4/1 -> Saturation3/1
  Saturation3/1 -> Divide1/2
  Te_ref/1 -> Divide1/1
  Grid/1 -> Bus Selector2/1
  Bus Selector1/2 -> Add1/1  "<q>"
  Bus Selector2/1 -> Add1/2  "<Qs_ref>"

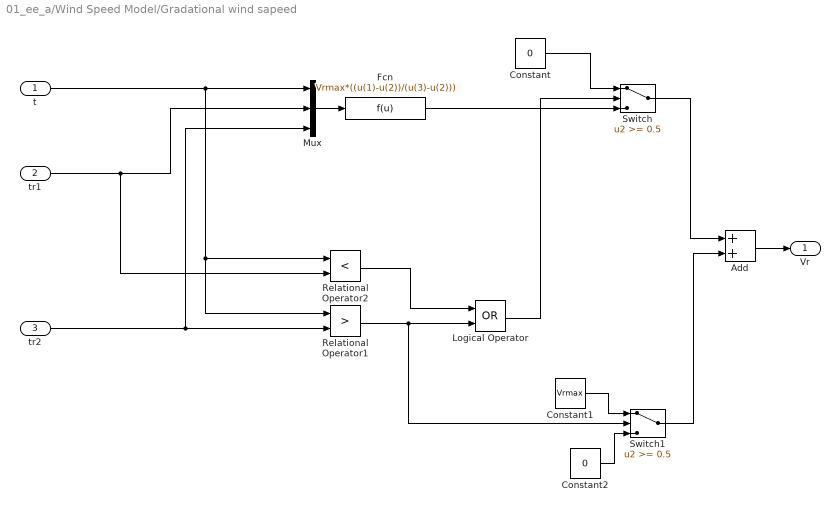
== system 01_ee_a/Wind Speed Model/Gradational wind sapeed ==
  t : Inport
  tr1 : Inport  Port=2
  tr2 : Inport  Port=3
  Add : Sum
  Constant : Constant  Value=0
  Constant1 : Constant  Value=Vrmax
  Constant2 : Constant  Value=0
  Fcn : Fcn  Expr=Vrmax*((u(1)-u(2))/(u(3)-u(2)))
  Logical Operator : Logic  Operator=OR  AllPortsSameDT=off  OutDataTypeStr=boolean
  Mux : Mux  Inputs=3
  Relational Operator1 : RelationalOperator  Operator=>  OutDataTypeStr=boolean  InputSameDT=off
  Relational Operator2 : RelationalOperator  Operator=<  OutDataTypeStr=boolean  InputSameDT=off
  Switch : Switch  Threshold=0.5  SaturateOnIntegerOverflow=off  InputSameDT=off
  Switch1 : Switch  Threshold=0.5  SaturateOnIntegerOverflow=off  InputSameDT=off
  Vr : Outport
  wires:
  Mux/1 -> Fcn/1
  tr1/1 -> Mux/2, Relational Operator2/2
  t/1 -> Mux/1, Relational Operator2/1, Relational Operator1/1
  tr2/1 -> Relational Operator1/2, Mux/3
  Relational Operator2/1 -> Logical Operator/1
  Relational Operator1/1 -> Switch1/2, Logical Operator/2
  Logical Operator/1 -> Switch/2
  Constant/1 -> Switch/1
  Fcn/1 -> Switch/3
  Switch/1 -> Add/1
  Switch1/1 -> Add/2
  Add/1 -> Vr/1
  Constant2/1 -> Switch1/3
  Constant1/1 -> Switch1/1

== system 01_ee_a/Wind Speed Model/Turbulent wind speed  ==
  t : Inport
  tg1 : Inport  Port=2
  Tg : Inport  Port=3
  Add : Sum
  Constant : Constant  Value=0
  Fcn : Fcn  Expr=0.5*Vgmax*(1-cos(2*pi*(u(1)-u(2))/u(3)))
  Logical Operator : Logic  Operator=OR  AllPortsSameDT=off  OutDataTypeStr=boolean
  Mux : Mux  Inputs=3
  Relational Operator1 : RelationalOperator  Operator=>  OutDataTypeStr=boolean  InputSameDT=off
  Relational Operator2 : RelationalOperator  Operator=<  OutDataTypeStr=boolean  InputSameDT=off
  Switch : Switch  Threshold=0.5  SaturateOnIntegerOverflow=off  InputSameDT=off
  Vg : Outport
  wires:
  t/1 -> Mux/1, Relational Operator2/1, Relational Operator1/1
  tg1/1 -> Mux/2, Add/1, Relational Operator2/2
  Mux/1 -> Fcn/1
  Switch/1 -> Vg/1
  Relational Operator2/1 -> Logical Operator/1
  Relational Operator1/1 -> Logical Operator/2
  Logical Operator/1 -> Switch/2
  Fcn/1 -> Switch/3
  Constant/1 -> Switch/1
  Add/1 -> Relational Operator1/2
  Tg/1 -> Mux/3, Add/2

== system 01_ee_a/Wind Turbine Control system/MPPT ==
  wr : Inport
  Grid : Inport  Port=2
  Add2 : Sum
  Bus Selector1 : BusSelector  OutputSignals=Max Power
  Divide2 : Product  Inputs=*/
  Fcn : Fcn  Expr=u^3
  Gain : Gain  Gain=1/(1.1)^3
  P_loss : Constant  Value=0
  Saturation1 : Saturate  UpperLimit=1.3  LowerLimit=0.1
  Switch : Switch  Threshold=1.1  SaturateOnIntegerOverflow=off  InputSameDT=off
  Te_ref : Outport
  wires:
  Fcn/1 -> Gain/1
  Gain/1 -> Add2/1
  P_loss/1 -> Add2/2
  wr/1 -> Fcn/1, Saturation1/1, Switch/2
  Add2/1 -> Switch/3
  Switch/1 -> Divide2/1  "P_ref"
  Saturation1/1 -> Divide2/2
  Divide2/1 -> Te_ref/1  "T_ref"
  Grid/1 -> Bus Selector1/1
  Bus Selector1/1 -> Switch/1  "<Max Power>"

== system 01_ee_a/Wind Turbine Control system/Pitch control ==
  wr : Inport
  0-pitch_max : Saturate  UpperLimit=45  LowerLimit=0
  Constant2 : Constant  Value=1.2
  "Rate Limiter   " : RateLimiter  RisingSlewLimit=2  FallingSlewLimit=-2
  Sum : Sum  Inputs=|+-  SaturateOnIntegerOverflow=on
  pitch_gain : Gain  Gain=500  SaturateOnIntegerOverflow=on  OutDataTypeStr=Inherit: Same as input  ParamDataTypeStr=Inherit: Same as input
  Pitch angle : Outport
  wires:
  wr/1 -> Sum/1
  "Rate Limiter   "/1 -> Pitch angle/1
  pitch_gain/1 -> 0-pitch_max/1
  Sum/1 -> pitch_gain/1
  Constant2/1 -> Sum/2
  0-pitch_max/1 -> "Rate Limiter   "/1

== system 01_ee_a/Data acquisition/Active & Reactive Power/Filter ==
  p_q : Inport
  Bus Creator : BusCreator  Inputs=2
  Constant : Constant  Value=fnom
  Demux2 : Demux  Outputs=2
  Discrete Variable Frequency Mean value : powerlib_extras/Discrete Measurements/Discrete Variable Frequency Mean value  Finit=50  Fmin=45  Vinit=0  Ts=Ts_Power
  Discrete Variable Frequency Mean value1 : powerlib_extras/Discrete Measurements/Discrete Variable Frequency Mean value  Finit=50  Fmin=45  Vinit=0  Ts=Ts_Power
  P_Q_Average : Outport
  wires:
  Constant/1 -> Discrete Variable Frequency Mean value/1, Discrete Variable Frequency Mean value1/1
  Discrete Variable Frequency Mean value/1 -> Bus Creator/1  "P"
  Discrete Variable Frequency Mean value1/1 -> Bus Creator/2  "Q"
  Demux2/1 -> Discrete Variable Frequency Mean value/2
  Demux2/2 -> Discrete Variable Frequency Mean value1/2
  Bus Creator/1 -> P_Q_Average/1
  p_q/1 -> Demux2/1

== system 01_ee_a/Data acquisition/Active & Reactive Power/Low pass filter ==
  p_q : Inport
  Bus Creator : BusCreator  Inputs=2
  Demux2 : Demux  Outputs=2
  Discrete 2nd-Order Filter1 : powerlib_extras/Discrete  Control Blocks/Discrete  2nd-Order Filter  FilterType=Lowpass  Fo=200  Zeta=0.707  Ts=Ts_Power  Initialize=off  Vac_Init=[0.8 -25 60]  Vdc_Init=-0.4  PlotResponse=off  param1=[1 500 1]
  Discrete 2nd-Order Filter2 : powerlib_extras/Discrete  Control Blocks/Discrete  2nd-Order Filter  FilterType=Lowpass  Fo=200  Zeta=0.707  Ts=Ts_Power  Initialize=off  Vac_Init=[0.8 -25 60]  Vdc_Init=-0.4  PlotResponse=off  param1=[1 500 1]
  "p_q_Transient " : Outport
  wires:
  Discrete 2nd-Order Filter2/1 -> Bus Creator/1  "p"
  Discrete 2nd-Order Filter1/1 -> Bus Creator/2  "q"
  Demux2/1 -> Discrete 2nd-Order Filter2/1
  Demux2/2 -> Discrete 2nd-Order Filter1/1
  p_q/1 -> Demux2/1
  Bus Creator/1 -> "p_q_Transient "/1

== system 01_ee_a/Data acquisition/Transformation abc --> dq /(-2pi 2pi) to (0 2pi) ==
  In : Inport
  Add : Sum
  Constant : Constant  Value=2*pi
  Switch : Switch  SaturateOnIntegerOverflow=off  InputSameDT=off
  Out : Outport
  wires:
  In/1 -> Switch/2, Switch/1, Add/1
  Constant/1 -> Add/2
  Add/1 -> Switch/3
  Switch/1 -> Out/1

== system 01_ee_a/Data acquisition/Transformation abc --> dq /abc_to_dq ==
  abc : Inport
  sin_cos : Inport  Port=2
  Bus Creator : BusCreator  Inputs=2
  Demux7 : Demux  Outputs=3
      settings: DisplayOption=none
  Terminator6 : Terminator
  abc_to_dq0 3 : powerlib_extras/Measurements/abc_to_dq0 Transformation
  dq : Outport
  wires:
  sin_cos/1 -> abc_to_dq0 3/2
  abc/1 -> abc_to_dq0 3/1
  abc_to_dq0 3/1 -> Demux7/1
  Demux7/3 -> Terminator6/1
  Bus Creator/1 -> dq/1
  Demux7/1 -> Bus Creator/1  "d"
  Demux7/2 -> Bus Creator/2  "q"

== system 01_ee_a/Data acquisition/Transformation abc --> dq /abc_to_dq1 ==
  abc : Inport
  sin_cos : Inport  Port=2
  Bus Creator : BusCreator  Inputs=2
  Demux7 : Demux  Outputs=3
      settings: DisplayOption=none
  Terminator6 : Terminator
  abc_to_dq0 3 : powerlib_extras/Measurements/abc_to_dq0 Transformation
  dq : Outport
  wires:
  Demux7/2 -> Bus Creator/2  "q"
  Demux7/1 -> Bus Creator/1  "d"
  Bus Creator/1 -> dq/1
  Demux7/3 -> Terminator6/1
  abc_to_dq0 3/1 -> Demux7/1
  abc/1 -> abc_to_dq0 3/1
  sin_cos/1 -> abc_to_dq0 3/2

== system 01_ee_a/Data acquisition/Transformation abc --> dq /abc_to_dq2 ==
  abc : Inport
  sin_cos : Inport  Port=2
  Bus Creator : BusCreator  Inputs=2
  Demux7 : Demux  Outputs=3
      settings: DisplayOption=none
  Terminator6 : Terminator
  abc_to_dq0 3 : powerlib_extras/Measurements/abc_to_dq0 Transformation
  dq : Outport
  wires:
  sin_cos/1 -> abc_to_dq0 3/2
  abc/1 -> abc_to_dq0 3/1
  abc_to_dq0 3/1 -> Demux7/1
  Demux7/3 -> Terminator6/1
  Bus Creator/1 -> dq/1
  Demux7/1 -> Bus Creator/1  "d"
  Demux7/2 -> Bus Creator/2  "q"

== system 01_ee_a/Data acquisition/Transformation abc --> dq /abc_to_dq3 ==
  abc : Inport
  Theta : Inport  Port=2
  Bus Creator : BusCreator  Inputs=2
  Demux7 : Demux  Outputs=3
      settings: DisplayOption=none
  Mux6 : Mux  Inputs=2
  Terminator6 : Terminator
  Trigonometric Function11 : Trigonometry
  Trigonometric Function12 : Trigonometry  Operator=cos
  abc_to_dq0 3 : powerlib_extras/Measurements/abc_to_dq0 Transformation
  dq : Outport
  wires:
  abc_to_dq0 3/1 -> Demux7/1
  Mux6/1 -> abc_to_dq0 3/2
  abc/1 -> abc_to_dq0 3/1
  Trigonometric Function11/1 -> Mux6/1
  Trigonometric Function12/1 -> Mux6/2
  Theta/1 -> Trigonometric Function11/1, Trigonometric Function12/1
  Demux7/3 -> Terminator6/1
  Bus Creator/1 -> dq/1
  Demux7/1 -> Bus Creator/1  "d"
  Demux7/2 -> Bus Creator/2  "q"

== system 01_ee_a/Grid Operators Control system/voltage control/Discrete PI Controller2 ==
  note: Discrete PID Controller
  note: Pierre Giroux, Gilbert Sybille
      | Power System Simulation Laboratory
      | IREQ, Hydro-Quebc
  Error : Inport
  Discrete-Time Integrator : DiscreteIntegrator  InitialCondition=Init  SampleTime=Ts  LimitOutput=on  UpperSaturationLimit=UpperLimit  LowerSaturationLimit=LowerLimit  ICPrevOutput=DiscIntNeverNeededParam  ICPrevScaledInput=DiscIntNeverNeededParam
  Kp4 : Gain  Gain=Kp  SaturateOnIntegerOverflow=on  OutDataTypeStr=Inherit: Same as input  ParamDataTypeStr=Inherit: Same as input
  Kp5 : Gain  Gain=Ki  SaturateOnIntegerOverflow=on  OutDataTypeStr=Inherit: Same as input  ParamDataTypeStr=Inherit: Same as input
  Saturation2 : Saturate  UpperLimit=UpperLimit  LowerLimit=LowerLimit
  Sum6 : Sum  InputSameDT=on  SaturateOnIntegerOverflow=on  OutDataTypeStr=Inherit: Same as first input
  Out : Outport  InitialOutput=0
  wires:
  Saturation2/1 -> Out/1
  Discrete-Time Integrator/1 -> Sum6/2
  Kp4/1 -> Sum6/1
  Kp5/1 -> Discrete-Time Integrator/1
  Sum6/1 -> Saturation2/1
  Error/1 -> Kp5/1, Kp4/1

== system 01_ee_a/Grid-side converter Control system/Current regulator/Discrete PI Controller1 ==
  note: Discrete PID Controller
  note: Pierre Giroux, Gilbert Sybille
      | Power System Simulation Laboratory
      | IREQ, Hydro-Quebc
  Error : Inport
  Discrete-Time Integrator : DiscreteIntegrator  InitialCondition=Init  SampleTime=Ts  LimitOutput=on  UpperSaturationLimit=UpperLimit  LowerSaturationLimit=LowerLimit  ICPrevOutput=DiscIntNeverNeededParam  ICPrevScaledInput=DiscIntNeverNeededParam
  Kp4 : Gain  Gain=Kp  SaturateOnIntegerOverflow=on  OutDataTypeStr=Inherit: Same as input  ParamDataTypeStr=Inherit: Same as input
  Kp5 : Gain  Gain=Ki  SaturateOnIntegerOverflow=on  OutDataTypeStr=Inherit: Same as input  ParamDataTypeStr=Inherit: Same as input
  Saturation2 : Saturate  UpperLimit=UpperLimit  LowerLimit=LowerLimit
  Sum6 : Sum  InputSameDT=on  SaturateOnIntegerOverflow=on  OutDataTypeStr=Inherit: Same as first input
  Waveforms : Scope  NumInputPorts=3
  Out : Outport  InitialOutput=0
  wires:
  Saturation2/1 -> Waveforms/3, Out/1
  Discrete-Time Integrator/1 -> Waveforms/2, Sum6/2
  Kp4/1 -> Waveforms/1, Sum6/1
  Kp5/1 -> Discrete-Time Integrator/1
  Sum6/1 -> Saturation2/1
  Error/1 -> Kp5/1, Kp4/1

== system 01_ee_a/Grid-side converter Control system/Current regulator/Discrete PI Controller2 ==
  note: Pierre Giroux, Gilbert Sybille
      | Power System Simulation Laboratory
      | IREQ, Hydro-Quebc
  note: Discrete PID Controller
  Error : Inport
  Discrete-Time Integrator : DiscreteIntegrator  InitialCondition=Init  SampleTime=Ts  LimitOutput=on  UpperSaturationLimit=UpperLimit  LowerSaturationLimit=LowerLimit  ICPrevOutput=DiscIntNeverNeededParam  ICPrevScaledInput=DiscIntNeverNeededParam
  Kp4 : Gain  Gain=Kp  SaturateOnIntegerOverflow=on  OutDataTypeStr=Inherit: Same as input  ParamDataTypeStr=Inherit: Same as input
  Kp5 : Gain  Gain=Ki  SaturateOnIntegerOverflow=on  OutDataTypeStr=Inherit: Same as input  ParamDataTypeStr=Inherit: Same as input
  Saturation2 : Saturate  UpperLimit=UpperLimit  LowerLimit=LowerLimit
  Sum6 : Sum  InputSameDT=on  SaturateOnIntegerOverflow=on  OutDataTypeStr=Inherit: Same as first input
  Out : Outport  InitialOutput=0
  wires:
  Error/1 -> Kp4/1, Kp5/1
  Sum6/1 -> Saturation2/1
  Kp5/1 -> Discrete-Time Integrator/1
  Kp4/1 -> Sum6/1
  Discrete-Time Integrator/1 -> Sum6/2
  Saturation2/1 -> Out/1

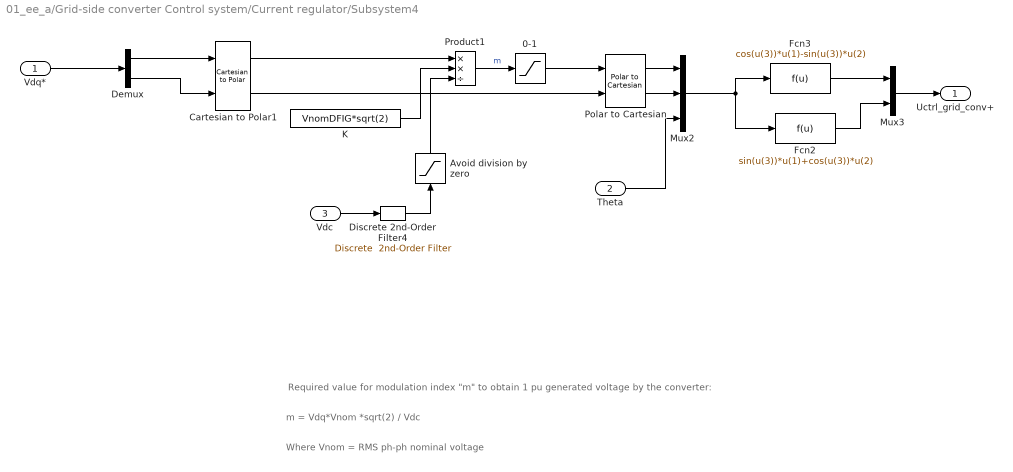
== system 01_ee_a/Grid-side converter Control system/Current regulator/Subsystem4 ==
  note: Required value for modulation index "m" to obtain 1 pu generated voltage by the converter:
  note: m = Vdq*Vnom *sqrt(2) / Vdc
  note: Where Vnom = RMS ph-ph nominal voltage
  Vdq* : Inport
  Theta : Inport  Port=2
  Vdc : Inport  Port=3
  0-1 : Saturate  UpperLimit=1  LowerLimit=0
  Avoid division by zero : Saturate  UpperLimit=1e5  LowerLimit=10
  Cartesian to Polar1 : simulink_extras/Transformations/Cartesian to Polar
  Demux : Demux  Outputs=2
  Discrete 2nd-Order Filter4 : powerlib_extras/Discrete  Control Blocks/Discrete  2nd-Order Filter  FilterType=Lowpass  Fo=50  Zeta=0.707  Ts=Ts_Power  Initialize=off  Vac_Init=[0.8 -25 60]  Vdc_Init=-0.4  PlotResponse=off  param1=[1 5000 10]
  Fcn2 : Fcn  Expr=sin(u(3))*u(1)+cos(u(3))*u(2)  SampleTime=Ts_Power
  Fcn3 : Fcn  Expr=cos(u(3))*u(1)-sin(u(3))*u(2)  SampleTime=Ts_Power
  K : Constant  Value=VnomDFIG*sqrt(2)
  Mux2 : Mux  Inputs=3
  Mux3 : Mux  Inputs=2
  Polar to Cartesian : simulink_extras/Transformations/Polar to Cartesian
  Product1 : Product  Inputs=**/  InputSameDT=on  SaturateOnIntegerOverflow=on  OutDataTypeStr=Inherit: Same as first input
  Uctrl_grid_conv+ : Outport
  wires:
  Mux3/1 -> Uctrl_grid_conv+/1
  Fcn3/1 -> Mux3/1
  Fcn2/1 -> Mux3/2
  Demux/1 -> Cartesian to Polar1/1
  Demux/2 -> Cartesian to Polar1/2
  0-1/1 -> Polar to Cartesian/1
  Product1/1 -> 0-1/1  "m"
  Vdc/1 -> Discrete 2nd-Order Filter4/1
  K/1 -> Product1/2
  Avoid division by zero/1 -> Product1/3
  Cartesian to Polar1/1 -> Product1/1
  Cartesian to Polar1/2 -> Polar to Cartesian/2
  Vdq*/1 -> Demux/1
  Polar to Cartesian/1 -> Mux2/1
  Polar to Cartesian/2 -> Mux2/2
  Theta/1 -> Mux2/3
  Mux2/1 -> Fcn3/1, Fcn2/1
  Discrete 2nd-Order Filter4/1 -> Avoid division by zero/1
